simulink model "bonus_model"  (R2021b)
settings: Solver=VariableStepAuto  StartTime=0.0  StopTime=2  RelTol=1e-3
values from neighbouring files (symbols this model uses):
  AmpDen = [1 655.7 5.52e6]    [draft_model_variables.m]    (also in linear_model_variables.m = [1 655.7 7.704e5])
  AmpNum = [2.149e7]    [draft_model_variables.m]    (also in linear_model_variables.m = [3e06])
  CF = 1000    [derivative_filter.m]    (also in draft_model_variables.m = 1163; linear_model_variables.m = 10000)
  K1 = 0.589    [draft_model_variables.m]
  K2 = 0.0753    [draft_model_variables.m]
  Kd1 = 109.6356    [draft_model_variables.m]    (also in linear_model_variables.m = 3)
  Kd2 = 99.9905    [draft_model_variables.m]    (also in linear_model_variables.m = 2)
  Ki1 = 1    [draft_model_variables.m]    (also in linear_model_variables.m = 0)
  Ki2 = 1    [draft_model_variables.m]    (also in linear_model_variables.m = 0)
  Kp1 = 20.9419    [draft_model_variables.m]    (also in linear_model_variables.m = 2)
  Kp2 = 19.9995    [draft_model_variables.m]    (also in linear_model_variables.m = 1)
  N = 10    [derivative_filter.m]    (also in draft_model_variables.m = 100)
  s = tf('s')    [draft_model_variables.m]
undefined symbols (not defined in the file or in its folder): gear1, gear2, gear3, K3, ka1, ka2, ka3, Kd3, Ki3, km1, km2, km3, Kp3, L1, L2, L3, R1, R2, R3
libraries: cstblocks x3, simulink x3
settings Model: Creator=ncamp  LastModifiedBy=ncamp

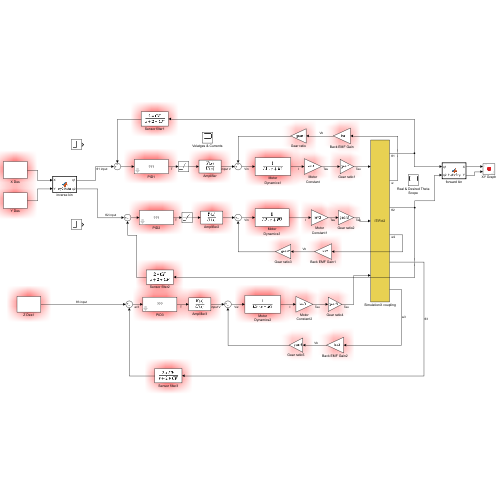
[thumbnail: Simulink's stored preview of the top-level diagram]
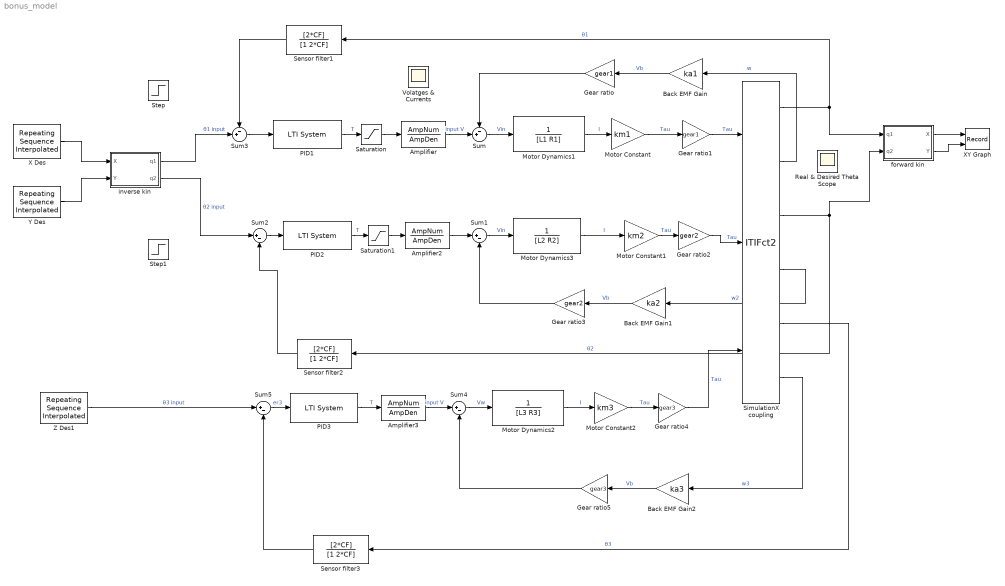
== system bonus_model ==
  Amplifier : TransferFcn  Numerator=AmpNum  Denominator=AmpDen
  Amplifier2 : TransferFcn  Numerator=AmpNum  Denominator=AmpDen
  Amplifier3 : TransferFcn  Numerator=AmpNum  Denominator=AmpDen
  Back EMF Gain : Gain  Gain=ka1
  Back EMF Gain1 : Gain  Gain=ka2
  Back EMF Gain2 : Gain  Gain=ka3
  Gear ratio : Gain  Gain=gear1
  Gear ratio1 : Gain  Gain=gear1
  Gear ratio2 : Gain  Gain=gear2
  Gear ratio3 : Gain  Gain=gear2
  Gear ratio4 : Gain  Gain=gear3
  Gear ratio5 : Gain  Gain=gear3
  Motor Constant : Gain  Gain=km1
  Motor Constant1 : Gain  Gain=km2
  Motor Constant2 : Gain  Gain=km3
  Motor Dynamics1 : TransferFcn  Denominator=[L1 R1]
  Motor Dynamics2 : TransferFcn  Denominator=[L3 R3]
  Motor Dynamics3 : TransferFcn  Denominator=[L2 R2]
  PID1 : cstblocks/LTI System  sys=tf(K1*Kp1 + K1*Ki1/s + K1*Kd1*N*s/(s+N))  IC=[]
  PID2 : cstblocks/LTI System  sys=tf(K2*Kp2 + K2*Ki2/s + K2*Kd2*N*s/(s+N))  IC=[]
  PID3 : cstblocks/LTI System  sys=tf(K3*Kp3 + K3*Ki3/s + K3*Kd3*N*s/(s+N))  IC=[]
  Real & Desired Theta Scope : Scope
      settings: Floating=on
  Saturation : Saturate  UpperLimit=5  LowerLimit=-5
  Saturation1 : Saturate  UpperLimit=5  LowerLimit=-5
  Sensor filter1 : TransferFcn  Numerator=[2*CF]  Denominator=[1 2*CF]
  Sensor filter2 : TransferFcn  Numerator=[2*CF]  Denominator=[1 2*CF]
  Sensor filter3 : TransferFcn  Numerator=[2*CF]  Denominator=[1 2*CF]
  SimulationX coupling : S-Function  FunctionName=ITIFct2  Parameters=ip, port, ts, nIn, nOut  SFunctionDeploymentMode=off  EnableBusSupport=off  mask{ip='localhost', port=4097, ts=0.001, nIn=3, nOut=6}
      mask prompts: ip "Address: ip"; port "Port Number: port [-]"; ts "Communication Step Size: ts [s]"; nIn "Input Vector Dimension (to SimulationX): nIn [-]"; nOut "Output Vector Dimension (from SimulationX): nOut [-]"
      mask help: Coupling Element
  Step : Step  After=0.01  SampleTime=0
  Step1 : Step  Time=0.1  After=0.01  SampleTime=0
  Sum : Sum  Inputs=-+|
  Sum{1..2,4..5} (4 alike) : Sum  Inputs=|+-
  Sum3 : Sum  Inputs=-+|
  Volatges & Currents : Scope
      settings: Floating=on
  X Des : simulink/Sources/Repeating Sequence Interpolated  OutValues=X  TimeValues=time  LookUpMeth=Interpolation-Use End Values  tsamp=0.001  OutMin=[]  OutMax=[]  OutDataTypeStr=double  OutputDataTypeScalingMode=double  OutDataType=fixdt(0,8)  OutScaling=2^-10
  XY Graph : Record  FileSettingsInternal="{\"entries\":[{\"content\":{\"excelSettings\":{\"content\":{},\"type\":\"Streamout.ExcelSettings\"}},\"type\":\"Streamout.FileSettingStorage\",\"uuid\":\"8784a271-8f35-4e30-9e53-f6e411d4ccb4\"}],\"packageUris\":[\"http://schema.mathworks.com/mf0/streamout_blocks/R2020a\"],\"version\":\"1.0\"}"  Layout=[1 2]  SignalsInternal="{\"entries\":[{\"content\":{\"signals\":[{\"content\":{\"blockPath\":[\"draft_arm_model/XY Graph\"],\"channel\":[],\"dimensions\":[1],\"domain\":\"draft_arm_model/XY Graph\",\"lineColor\":\"#ff13a6\",\"plots\":[],\"port\":1,\"sid\":[],\"signalID\":1541,\"signalName\":\"forward kin:1\"},\"type\":\"RecordBlkView.Signal\",\"uuid\":\"780cc8cf-f642-4b40-8978-12698b9b9794\"},{\"content\":{\"blockPath\":[\"draft_arm_model/XY Graph\"],\"channel\":[],\"dimensions\":[1],\"domain\":\"draft_arm_model/XY Graph\",\"lineColor\":\"#fe330a\",\"plots\":[],\"port\":2,\"sid\":[],\"signalID\":1544,\"signalName\":\"forward kin:2\"},\"type\":\"RecordBlkView.Signal\",\"uuid\":\"c3f45100-836b-4b3a-96e9-61f07f065cd6\"}]},\"type\":\"RecordBlkView.InputSignals\",\"uuid\":\"ad2cb79a-d5ca-4cf1-bcf8-d717a850ceee\"}],\"packageUris\":[\"http://schema.mathworks.com/mf0/streamout_blocks/R2020a\"],\"version\":\"1.0\"}"  VisualizationBindings="{\"xyplotplugin\":{\"info\":[{\"series\":[],\"subplotID\":1}]}}"  CompatibilityTag=XY
  Y Des : simulink/Sources/Repeating Sequence Interpolated  OutValues=Y  TimeValues=time  LookUpMeth=Interpolation-Use End Values  tsamp=0.001  OutMin=[]  OutMax=[]  OutDataTypeStr=double  OutputDataTypeScalingMode=double  OutDataType=fixdt(0,8)  OutScaling=2^-10
  Z Des1 : simulink/Sources/Repeating Sequence Interpolated  OutValues=Z  TimeValues=time  LookUpMeth=Interpolation-Use End Values  tsamp=0.001  OutMin=[]  OutMax=[]  OutDataTypeStr=double  OutputDataTypeScalingMode=double  OutDataType=fixdt(0,8)  OutScaling=2^-10
  forward kin : MATLAB Function  TreatAsAtomicUnit=on
  inverse kin : MATLAB Function  TreatAsAtomicUnit=on
  wires:
  Back EMF Gain/1 -> Gear ratio/1  "Vb"
  Motor Dynamics1/1 -> Motor Constant/1  "I"
  Sum/1 -> Motor Dynamics1/1  "Vin"
  Back EMF Gain1/1 -> Gear ratio3/1  "Vb"
  Motor Dynamics3/1 -> Motor Constant1/1  "I"
  Sum1/1 -> Motor Dynamics3/1  "Vin"
  Sum2/1 -> PID2/1
  inverse kin/2(q2) -> Sum2/1  "θ2 input"
  PID2/1 -> Saturation1/1  "T"
  Amplifier2/1 -> Sum1/1
  PID1/1 -> Saturation/1  "T"
  Amplifier/1 -> Sum/2  "input V"
  inverse kin/1(q1) -> Sum3/2  "θ1 input"
  Sum3/1 -> PID1/1
  Motor Constant1/1 -> Gear ratio2/1  "Tau"
  Gear ratio2/1 -> SimulationX coupling/2  "Tau"
  Motor Constant/1 -> Gear ratio1/1  "Tau"
  Gear ratio1/1 -> SimulationX coupling/1  "Tau"
  Gear ratio3/1 -> Sum1/2
  Gear ratio/1 -> Sum/1
  SimulationX coupling/2 -> Back EMF Gain/1  "w"
  SimulationX coupling/1 -> forward kin/1(q1), Sensor filter1/1  "θ1"
  SimulationX coupling/4 -> Back EMF Gain1/1  "w2"
  SimulationX coupling/3 -> Sensor filter2/1, forward kin/2(q2)  "θ2"
  forward kin/1(X) -> XY Graph/1
  forward kin/2(Y) -> XY Graph/2
  X Des/1 -> inverse kin/1(X)
  Y Des/1 -> inverse kin/2(Y)
  Sensor filter2/1 -> Sum2/2
  Sensor filter1/1 -> Sum3/1
  Saturation/1 -> Amplifier/1
  Saturation1/1 -> Amplifier2/1
  Gear ratio5/1 -> Sum4/2
  Sensor filter3/1 -> Sum5/2
  Back EMF Gain2/1 -> Gear ratio5/1  "Vb"
  Gear ratio4/1 -> SimulationX coupling/3  "Tau"
  SimulationX coupling/5 -> Sensor filter3/1  "θ3"
  Sum5/1 -> PID3/1  "er3"
  Motor Dynamics2/1 -> Motor Constant2/1  "I"
  Motor Constant2/1 -> Gear ratio4/1  "Tau"
  SimulationX coupling/6 -> Back EMF Gain2/1  "w3"
  PID3/1 -> Amplifier3/1  "T"
  Sum4/1 -> Motor Dynamics2/1  "Vw"
  Z Des1/1 -> Sum5/1  "θ3 input"
  Amplifier3/1 -> Sum4/1  "input V"

== matlab function bonus_model/inverse kin ==
  data: X input; q1 output; Y input; q2 output
function [q1,q2] = xy2theta(X,Y)

% Inputs X,Y should be in mm
% Outputs q1, q2 are in rads

L1 = 275;   % Arm 1 length (mm)
L2 = 275;   % Arm 2 length (mm)

% Elbow down position
q1 = 2*atan((2*L1*Y - (- L1^4 + 2*L1^2*L2^2 + 2*L1^2*X^2 + 2*L1^2*Y^2 - L2^4 + 2*L2^2*X^2 + 2*L2^2*Y^2 - X^4 - 2*X^2*Y^2 - Y^4)^(1/2))/(L1^2 + 2*L1*X - L2^2 + X^2 + Y^2));
q2 =  2*atan(((- L1^2 + 2*L1*L2 - L2^2 + X^2 + Y^2)*(L1^2 + 2*L1*L2 + L2^2 - X^2 - Y^2))^(1/2)/(- L1^2 + 2*L1*L2 - L2^2 + X^2 + Y^2));


end

== matlab function bonus_model/forward kin ==
  data: q1 input; X output; q2 input; Y output
function [X,Y] = theta2xy(q1,q2)

L1 = 275;
L2 = 275;

X = L1*cos(q1) + L2*cos(q1 + q2);
Y = L1*sin(q1) + L2*sin(q1 + q2);

end
